simulink model "Simulink_model"  (R2024b)
settings: Solver=VariableStepAuto  StartTime=0.0  StopTime=80  RelTol=1e-3
values from neighbouring files (symbols this model uses):
  default_spacing = 10    [ACC_Script.m]
  max_ac = 2    [ACC_Script.m]
  min_ac = -3.5    [ACC_Script.m]
  pos_ego = 10    [ACC_Script.m]
  pos_lead = 50    [ACC_Script.m]
  time_gap = 1.3    [ACC_Script.m]
  Ts = 0.25    [ACC_Script.m]
  v_set = 26    [ACC_Script.m]
  vel_ego = 28    [ACC_Script.m]
  vel_lead = 26    [ACC_Script.m]
  verr_gain = 1.4    [ACC_Script.m]
  vx_gain = 5.42    [ACC_Script.m]
  xerr_gain = 0.06    [ACC_Script.m]
libraries: simulink_extras x2
settings Model: Creator=Sowmy  LastModifiedBy=arunm

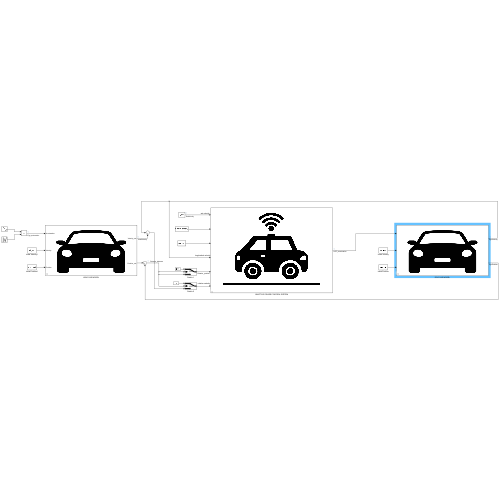
[thumbnail: Simulink's stored preview of the top-level diagram]
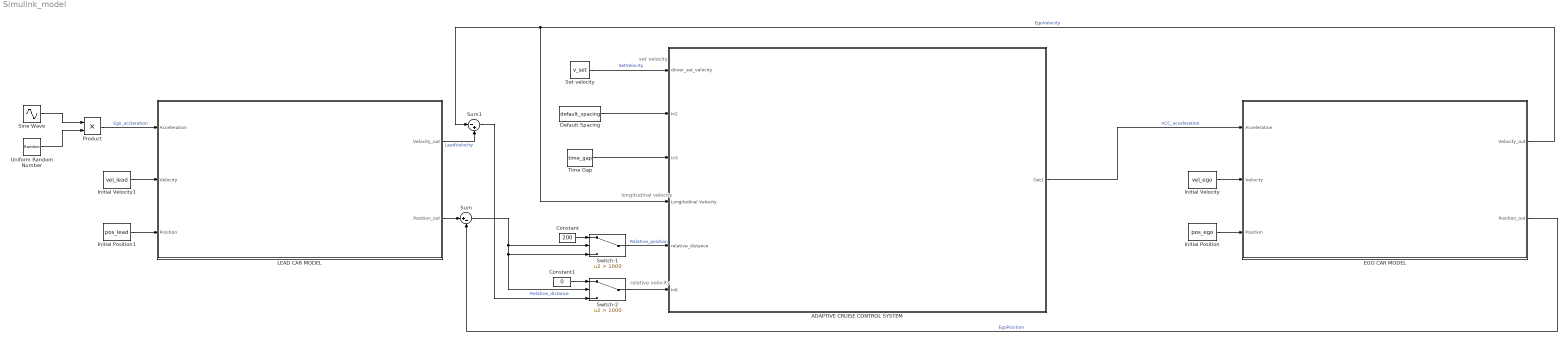
== system Simulink_model ==
  note: set velocity
  note: relative velocity
  note: longitudinal velocity
  ADAPTIVE CRUISE CONTROL SYSTEM : Subsystem
      mask Display: image("C:\CSE Project\AdobeStock_964843339.png");
  Constant : Constant  Value=200  SampleTime=-1
  Constant1 : Constant  Value=0  SampleTime=-1
  Default Spacing : Constant  Value=default_spacing  SampleTime=Ts
  EGO CAR MODEL : Subsystem
      mask Display: image("C:\CSE Project\CAR.jpg");
  Initial Position : Constant  Value=pos_ego  SampleTime=Ts
  Initial Position1 : Constant  Value=pos_lead  SampleTime=Ts
  Initial Velocity : Constant  Value=vel_ego  SampleTime=Ts
  Initial Velocity1 : Constant  Value=vel_lead  SampleTime=Ts
  LEAD CAR MODEL : Subsystem
      mask DialogControl Control2 Prompt: (Add text here)
      mask Display: image("C:\CSE Project\CAR.jpg");
  Product : Product
  Set velocity : Constant  Value=v_set  SampleTime=Ts
  Sine Wave : Sin  Amplitude=0.6  Frequency=0.1  SampleTime=Ts
  Sum : Sum  Inputs=|+-
  Sum1 : Sum  Inputs=|-+
  Switch-1 : Switch  Criteria=u2 > Threshold  Threshold=1000  SaturateOnIntegerOverflow=off  InputSameDT=off
  Switch-2 : Switch  Criteria=u2 > Threshold  Threshold=1000  SaturateOnIntegerOverflow=off  InputSameDT=off
  Time Gap : Constant  Value=time_gap  SampleTime=Ts
  Uniform Random Number : UniformRandomNumber  Minimum=-0.5  Maximum=0.5  SampleTime=Ts
  wires:
  ADAPTIVE CRUISE CONTROL SYSTEM/1(Out1) -> EGO CAR MODEL/1(Acceleration)  "ACC_acceleration"
  Initial Velocity/1 -> EGO CAR MODEL/2(Velocity)
  Initial Position/1 -> EGO CAR MODEL/3(Position)
  EGO CAR MODEL/2(Position_out) -> Sum/2  "EgoPosition"
  Default Spacing/1 -> ADAPTIVE CRUISE CONTROL SYSTEM/2(In2)
  EGO CAR MODEL/1(Velocity_out) -> ADAPTIVE CRUISE CONTROL SYSTEM/4(Longitudinal Velocity), Sum1/1  "EgoVelocity"
  Set velocity/1 -> ADAPTIVE CRUISE CONTROL SYSTEM/1(driver_set_velocity)  "SetVelocity"
  Time Gap/1 -> ADAPTIVE CRUISE CONTROL SYSTEM/3(In3)
  Initial Velocity1/1 -> LEAD CAR MODEL/2(Velocity)
  Initial Position1/1 -> LEAD CAR MODEL/3(Position)
  LEAD CAR MODEL/2(Position_out) -> Sum/1
  LEAD CAR MODEL/1(Velocity_out) -> Sum1/2  "LeadVelocity"
  Constant/1 -> Switch-1/1
  Constant1/1 -> Switch-2/1
  Sum/1 -> Switch-2/2, Switch-1/3, Switch-1/2  "Relative_distance"
  Switch-1/1 -> ADAPTIVE CRUISE CONTROL SYSTEM/5(relative_distance)  "Relative_position"
  Sum1/1 -> Switch-2/3
  Switch-2/1 -> ADAPTIVE CRUISE CONTROL SYSTEM/6(In6)
  Uniform Random Number/1 -> Product/2
  Sine Wave/1 -> Product/1
  Product/1 -> LEAD CAR MODEL/1(Acceleration)  "Ego_accleration"

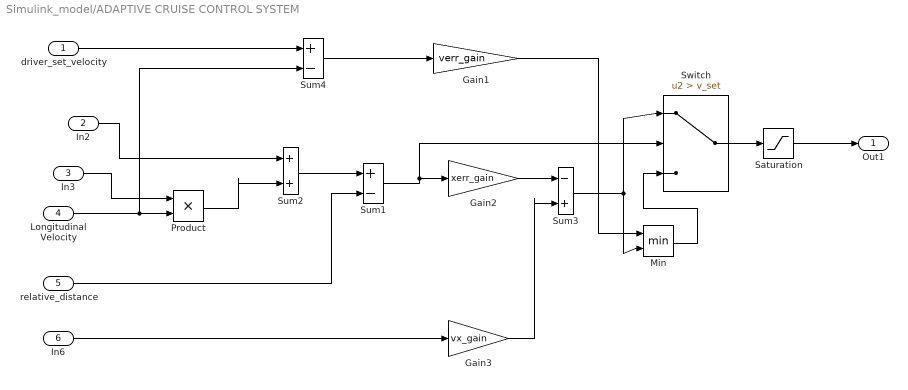
== system Simulink_model/ADAPTIVE CRUISE CONTROL SYSTEM ==
  driver_set_velocity : Inport
  In2 : Inport  Port=2
  In3 : Inport  Port=3
  Longitudinal Velocity : Inport  Port=4
  relative_distance : Inport  Port=5
  In6 : Inport  Port=6
  Gain1 : Gain  Gain=verr_gain
  Gain2 : Gain  Gain=xerr_gain
  Gain3 : Gain  Gain=vx_gain
  Min : MinMax  Inputs=2
  Product : Product
  Saturation : Saturate  UpperLimit=max_ac  LowerLimit=min_ac  RndMeth=Ceiling
  Sum1 : Sum  Inputs=+-
  Sum2 : Sum
  Sum3 : Sum  Inputs=-+
  Sum4 : Sum  Inputs=+-
  Switch : Switch  Criteria=u2 > Threshold  Threshold=v_set  SaturateOnIntegerOverflow=off  InputSameDT=off
  Out1 : Outport
  wires:
  Longitudinal Velocity/1 -> Product/2, Sum4/2
  Sum3/1 -> Min/2, Switch/1
  Gain1/1 -> Min/1
  Switch/1 -> Saturation/1
  Sum2/1 -> Sum1/1
  relative_distance/1 -> Sum1/2
  Sum4/1 -> Gain1/1
  Gain2/1 -> Sum3/1
  Min/1 -> Switch/3
  Product/1 -> Sum2/2
  Sum1/1 -> Switch/2, Gain2/1
  Gain3/1 -> Sum3/2
  In6/1 -> Gain3/1
  Saturation/1 -> Out1/1
  driver_set_velocity/1 -> Sum4/1
  In2/1 -> Sum2/1
  In3/1 -> Product/1

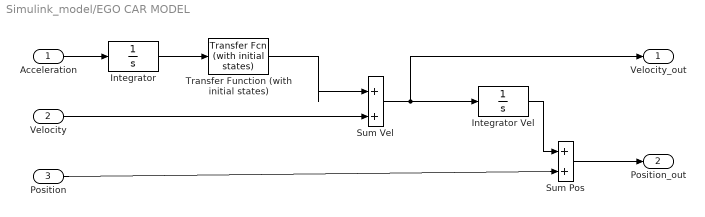
== system Simulink_model/EGO CAR MODEL ==
  Acceleration : Inport
  Velocity : Inport  Port=2
  Position : Inport  Port=3
  Integrator : Integrator
  Integrator Vel : Integrator
  Sum Pos : Sum  Inputs=|++
  Sum Vel : Sum  Inputs=|++
  Transfer Function (with initial states) : simulink_extras/Additional Linear/Transfer Fcn (with initial states)  N=[1]  D=[1 1]  X0=.5
  Velocity_out : Outport
  Position_out : Outport  Port=2
  wires:
  Integrator Vel/1 -> Sum Pos/1
  Velocity/1 -> Sum Vel/2
  Position/1 -> Sum Pos/2
  Integrator/1 -> Transfer Function (with initial states)/1
  Sum Vel/1 -> Velocity_out/1, Integrator Vel/1
  Transfer Function (with initial states)/1 -> Sum Vel/1
  Sum Pos/1 -> Position_out/1
  Acceleration/1 -> Integrator/1

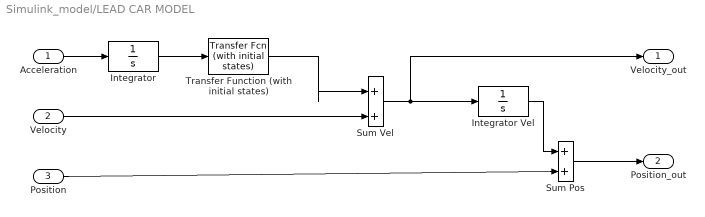
== system Simulink_model/LEAD CAR MODEL ==
  Acceleration : Inport  Description=Acceleration  SampleTime=Ts
  Velocity : Inport  Port=2
  Position : Inport  Port=3
  Integrator : Integrator
  Integrator Vel : Integrator
  Sum Pos : Sum  Inputs=|++
  Sum Vel : Sum  Inputs=|++
  Transfer Function (with initial states) : simulink_extras/Additional Linear/Transfer Fcn (with initial states)  N=[1]  D=[1 1 1]  X0=.5
  Velocity_out : Outport
  Position_out : Outport  Port=2
  wires:
  Integrator Vel/1 -> Sum Pos/1
  Velocity/1 -> Sum Vel/2
  Position/1 -> Sum Pos/2
  Integrator/1 -> Transfer Function (with initial states)/1
  Sum Vel/1 -> Velocity_out/1, Integrator Vel/1
  Transfer Function (with initial states)/1 -> Sum Vel/1
  Sum Pos/1 -> Position_out/1
  Acceleration/1 -> Integrator/1
